simulink model "Bang_bangControl"  (R2023b)
settings: Solver=VariableStepAuto  StartTime=0.0  StopTime=10.0  MaxStep=1e-4  RelTol=1e-3
values from neighbouring files (symbols this model uses):
  A = [0 1; 0 0]    [Bang_bang_init.m]
  B = [0;1]    [Bang_bang_init.m]
  C = eye(2)    [Bang_bang_init.m]
  D = zeros(2,1)    [Bang_bang_init.m]
  x_0 = [2 2]'    [Bang_bang_init.m]
settings Model: Creator=randolf  LastModifiedBy=randolf

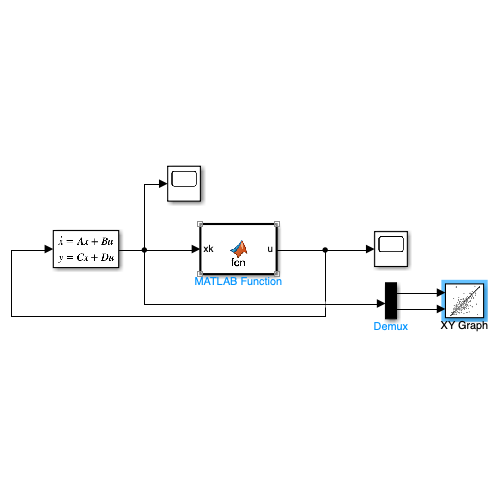
[thumbnail: Simulink's stored preview of the top-level diagram]
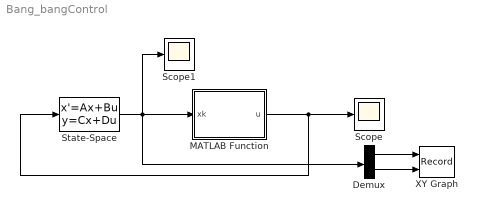
== system Bang_bangControl ==
  Demux : Demux  Outputs=2
  MATLAB Function : MATLAB Function  TreatAsAtomicUnit=on
  Scope : Scope
  Scope1 : Scope
  State-Space : StateSpace  A=A  B=B  C=C  D=D  InitialCondition=x_0
  XY Graph : Record  FileSettingsInternal="{\"entries\":[{\"content\":{\"excelSettings\":{\"content\":{},\"type\":\"Streamout.ExcelSettings\"}},\"type\":\"Streamout.FileSettingStorage\",\"uuid\":\"\"}],\"packageUris\":[\"http:\\/\\/schema.mathworks.com\\/mf0\\/streamout_blocks\\/R2020a\"],\"version\":\"1.0\"}"  Layout=[1 1]  SignalsInternal="{\"entries\":[{\"content\":{\"signals\":[{\"content\":{\"blockPath\":[],\"dimensions\":[1],\"domain\":\"\",\"lineColor\":\"#a2142f\",\"plots\":[1],\"port\":1,\"sid\":[\"\"],\"signalID\":35,\"signalName\":\"Demux:1\"},\"type\":\"RecordBlkView.Signal\",\"uuid\":\"\"},{\"content\":{\"blockPath\":[],\"dimensions\":[1],\"domain\":\"\",\"lineColor\":\"#139fff\",\"plots\":[1],\"port\":2,\"sid\":[\"\"],\"signalID\":39,\"signalName\":\"Demux:2\"},\"type\":\"RecordBlkView.Signal\",\"uuid\":\"\"}]},\"type\":\"RecordBlkView.InputSignals\",\"uuid\":\"\"}],\"packageUris\":[\"http:\\/\\/schema.mathworks.com\\/mf0\\/streamout_blocks\\/R2020a\"],\"version\":\"1.0\"}"  VisualizationBindings="{\"xyplotplugin\":{\"info\":[{\"series\":[{\"bindingParametersList\":[{\"parameter\":\"X-Axis\",\"signalID\":35,\"signalName\":\"Demux:1\"},{\"parameter\":\"Y-Axis\",\"signalID\":39,\"signalName\":\"Demux:2\"}],\"seriesID\":45400}],\"subplotID\":1}]}}"  CompatibilityTag=XY
  wires:
  State-Space/1 -> Demux/1, Scope1/1, MATLAB Function/1(xk)
  MATLAB Function/1(u) -> Scope/1, State-Space/1
  Demux/1 -> XY Graph/1
  Demux/2 -> XY Graph/2

== matlab function Bang_bangControl/MATLAB Function ==
  data: xk input; u output
function u  = fcn(xk)

    if   xk(1) <= -(1/2)*xk(2)*abs(xk(2))
        u = 1;
    else xk(1) >= -(1/2)*xk(2)*abs(xk(2))
        u = -1;
    end
end
